simulink model "singledof_demo"  (Simulink 7.8)
settings: Solver=FixedStepDiscrete  StartTime=0.0  StopTime=inf  FixedStep=Ts  RelTol=1e-3
PreLoadFcn:
  | loadParametersSingleDof
InitFcn:
  | loadParametersSingleDof
values from neighbouring files (symbols this model uses):
  L_arm = 0.075    [freemot.mat]    (also in loadParametersSingleDof.m)
  lowOrder_tfd_foh = c2d(tf([1 2*pi*.64154],[1 0]),Ts,'foh')    [loadParametersSingleDof.m]
  maxTorque_allowed = 1.125    [freemot.mat]    (also in loadParametersSingleDof.m)
  torque_constant = 3.112    [freemot.mat]    (also in loadParametersSingleDof.m)
  Ts = 0.0005    [freemot.mat]
undefined symbols (not defined in the file or in its folder): DiscIntNeverNeededParam, shuntDynPredict_part1_tfd_foh, shuntDynPredict_part2_tfd_foh
libraries: simulink x32, simulink_extras x3
(part 2 of 2)

== system singledof_demo/AO DO/LED ==
  note: groen slave
      | rood slave
      |
      | groen master
      | rood master
  Logical Operator{6,8..10} (4 alike) : Logic  Operator=OR  AllPortsSameDT=off  OutDataTypeStr=boolean
  Logical Operator11 : Logic  AllPortsSameDT=off  OutDataTypeStr=boolean
  Logical Operator2 : Logic  AllPortsSameDT=off  OutDataTypeStr=boolean
  Logical Operator7 : Logic  Operator=NOT  AllPortsSameDT=off  OutDataTypeStr=boolean
  Mux1 : Mux
  LED : Outport
  wires:
  [tau_dm_saturated] -> Logical Operator11/2
  Logical Operator11/1 -> Logical Operator8/2
  Logical Operator2/1 -> Logical Operator6/2
  [tau_rm_saturated] -> Logical Operator10/2
  [tau_rs_saturated] -> Logical Operator9/2
  Logical Operator10/1 -> Mux1/4
  Logical Operator9/1 -> Mux1/2
  Logical Operator8/1 -> Mux1/3
  Logical Operator7/1 -> Logical Operator10/1, Logical Operator8/1, Logical Operator9/1, Logical Operator6/1
  [init_complete] -> Logical Operator7/1
  Logical Operator6/1 -> Mux1/1
  [tau_ds_saturated] -> Logical Operator2/2
  [Passivity_enable] -> Logical Operator11/1, Logical Operator2/1
  Mux1/1 -> LED/1

== system singledof_demo/AO DO/extraSafety ==
  V1 : Inport
  V2 : Inport  Port=2
  Abs : Abs
  Abs1 : Abs
  Compare To Constant : simulink/Logic and Bit Operations/Compare To Constant  relop=>  const=.5  OutDataTypeStr=uint8
  Compare To Constant1 : simulink/Logic and Bit Operations/Compare To Constant  relop=>  const=.5  OutDataTypeStr=uint8
  Logical Operator : Logic  Operator=OR  AllPortsSameDT=off  OutDataTypeStr=boolean
  Stop Simulation : Stop
  wires:
  Compare To Constant1/1 -> Logical Operator/2
  Compare To Constant/1 -> Logical Operator/1
  V2/1 -> Abs1/1
  V1/1 -> Abs/1
  Logical Operator/1 -> Stop Simulation/1
  Abs1/1 -> Compare To Constant1/1
  Abs/1 -> Compare To Constant/1

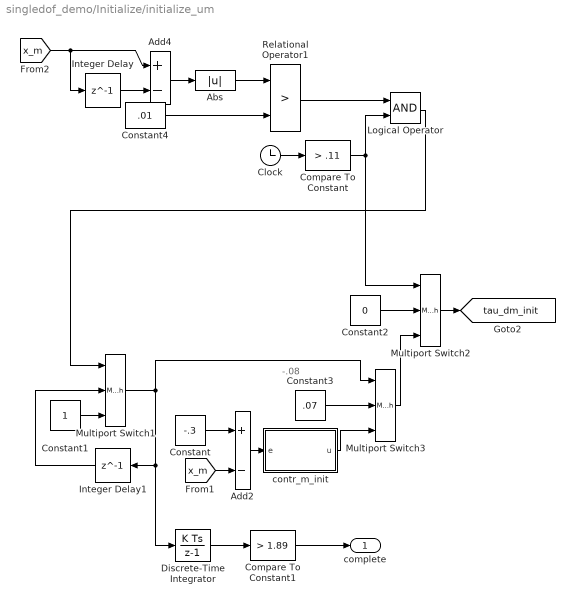
== system singledof_demo/Initialize/initialize_um ==
  note: -.08
  Abs : Abs
  Add2 : Sum  Inputs=+-
  Add4 : Sum  Inputs=+-
  Clock : Clock
  Compare To Constant : simulink/Logic and Bit Operations/Compare To Constant  relop=>  const=.11  OutDataTypeStr=uint8
  Compare To Constant1 : simulink/Logic and Bit Operations/Compare To Constant  relop=>  const=1.89  OutDataTypeStr=uint8
  Constant : Constant  Value=-.3
  Constant1 : Constant
  Constant2 : Constant  Value=0
  Constant3 : Constant  Value=.07
  Constant4 : Constant  Value=.01
  Discrete-Time Integrator : DiscreteIntegrator  SampleTime=Ts  ICPrevOutput=DiscIntNeverNeededParam  ICPrevScaledInput=DiscIntNeverNeededParam
  Integer Delay : Delay  DelayLength=1
  Integer Delay1 : Delay  DelayLength=1
  Logical Operator : Logic  AllPortsSameDT=off  OutDataTypeStr=boolean
  Multiport Switch1 : MultiPortSwitch  DataPortOrder=Zero-based contiguous  Inputs=2  zeroidx=on
  Multiport Switch2 : MultiPortSwitch  DataPortOrder=Zero-based contiguous  Inputs=2  zeroidx=on
  Multiport Switch3 : MultiPortSwitch  DataPortOrder=Zero-based contiguous  Inputs=2  zeroidx=on
  Relational Operator1 : RelationalOperator  Operator=>  OutDataTypeStr=boolean
  contr_m_init : Subsystem
      mask Display:
      | text(.1,.7,'Master')
      | text(.1,.3,'Controller')
  complete : Outport
  tag scope: tau_dm_init=global
  wires:
  Abs/1 -> Relational Operator1/1
  Constant2/1 -> Multiport Switch2/2
  Multiport Switch2/1 -> [tau_dm_init]
  Constant3/1 -> Multiport Switch3/2
  Multiport Switch3/1 -> Multiport Switch2/3
  contr_m_init/1(u) -> Multiport Switch3/3
  Compare To Constant1/1 -> complete/1
  Discrete-Time Integrator/1 -> Compare To Constant1/1
  Logical Operator/1 -> Multiport Switch1/1
  Compare To Constant/1 -> Multiport Switch2/1, Logical Operator/2
  Clock/1 -> Compare To Constant/1
  Relational Operator1/1 -> Logical Operator/1
  Add4/1 -> Abs/1
  [x_m] -> Integer Delay/1, Add4/1
  Constant4/1 -> Relational Operator1/2
  Integer Delay/1 -> Add4/2
  Constant/1 -> Add2/1
  Add2/1 -> contr_m_init/1(e)
  [x_m] -> Add2/2
  Constant1/1 -> Multiport Switch1/3
  Integer Delay1/1 -> Multiport Switch1/2
  Multiport Switch1/1 -> Multiport Switch3/1, Integer Delay1/1, Discrete-Time Integrator/1

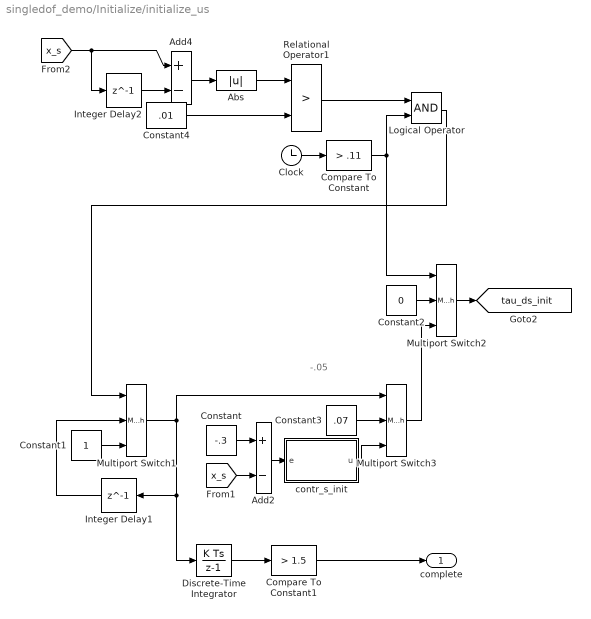
== system singledof_demo/Initialize/initialize_us ==
  note: -.05
  Abs : Abs
  Add2 : Sum  Inputs=+-
  Add4 : Sum  Inputs=+-
  Clock : Clock
  Compare To Constant : simulink/Logic and Bit Operations/Compare To Constant  relop=>  const=.11  OutDataTypeStr=uint8
  Compare To Constant1 : simulink/Logic and Bit Operations/Compare To Constant  relop=>  const=1.5  OutDataTypeStr=uint8
  Constant : Constant  Value=-.3
  Constant1 : Constant
  Constant2 : Constant  Value=0
  Constant3 : Constant  Value=.07
  Constant4 : Constant  Value=.01
  Discrete-Time Integrator : DiscreteIntegrator  SampleTime=Ts  ICPrevOutput=DiscIntNeverNeededParam  ICPrevScaledInput=DiscIntNeverNeededParam
  Integer Delay1 : Delay  DelayLength=1
  Integer Delay2 : Delay  DelayLength=1
  Logical Operator : Logic  AllPortsSameDT=off  OutDataTypeStr=boolean
  Multiport Switch1 : MultiPortSwitch  DataPortOrder=Zero-based contiguous  Inputs=2  zeroidx=on
  Multiport Switch2 : MultiPortSwitch  DataPortOrder=Zero-based contiguous  Inputs=2  zeroidx=on
  Multiport Switch3 : MultiPortSwitch  DataPortOrder=Zero-based contiguous  Inputs=2  zeroidx=on
  Relational Operator1 : RelationalOperator  Operator=>  OutDataTypeStr=boolean
  contr_s_init : Subsystem
      mask Display:
      | text(.1,.7,'Slave')
      | text(.1,.3,'Controller')
  complete : Outport
  tag scope: tau_ds_init=global
  wires:
  Abs/1 -> Relational Operator1/1
  Multiport Switch2/1 -> [tau_ds_init]
  Multiport Switch3/1 -> Multiport Switch2/3
  Constant2/1 -> Multiport Switch2/2
  contr_s_init/1(u) -> Multiport Switch3/3
  Constant3/1 -> Multiport Switch3/2
  Compare To Constant1/1 -> complete/1
  Discrete-Time Integrator/1 -> Compare To Constant1/1
  Multiport Switch1/1 -> Multiport Switch3/1, Integer Delay1/1, Discrete-Time Integrator/1
  Integer Delay1/1 -> Multiport Switch1/2
  Constant1/1 -> Multiport Switch1/3
  [x_s] -> Add2/2
  Add2/1 -> contr_s_init/1(e)
  Constant/1 -> Add2/1
  Integer Delay2/1 -> Add4/2
  Constant4/1 -> Relational Operator1/2
  [x_s] -> Integer Delay2/1, Add4/1
  Add4/1 -> Abs/1
  Relational Operator1/1 -> Logical Operator/1
  Clock/1 -> Compare To Constant/1
  Compare To Constant/1 -> Multiport Switch2/1, Logical Operator/2
  Logical Operator/1 -> Multiport Switch1/1

== system singledof_demo/Pos-force/contr_s ==
  e : Inport
  Add2 : Sum  Inputs=+++
  Discrete Derivative : simulink/Discrete/Discrete Derivative  gainval=1.0  ICPrevScaledInput=0.0  InputProcessing=Inherited  OutMin=[]  OutMax=[]  OutDataType=fixdt(1, 16)  OutScaling=2^-10  DoSatur=off
  Discrete-Time Integrator : DiscreteIntegrator  SampleTime=Ts  ICPrevOutput=DiscIntNeverNeededParam  ICPrevScaledInput=DiscIntNeverNeededParam
  Lowpass1 : Subsystem  mask{cf=100}
      mask prompts: cf "Cut off Frequency"
      mask help:
      | Discrete time first order lowpass filter, with cut-off frequency cf (Hz)
      | Kz / (z+K-1), with K=2*pi*cf*TS
      | For low frequencies this corresponds to the continous time lowpass filter
      | tf(1,[1/(2*pi*cf) 1])
      |
      | The maximum value for K=1, in this case output equals input
      | e.g. for 4000Hz sampling frequency the maximum value cf=4000/(2*pi)=637Hz.
      mask Display: text(.1,.5,['Lowpass @' num2str(cf) 'Hz'])
  P : Gain  Gain=Ps
  P1 : Gain  Gain=Is
  P2 : Gain  Gain=Ds
  anti windup : Subsystem
      mask Display: disp('anti-windup')
  u : Outport
  wires:
  Lowpass1/1(Out) -> P1/1, P2/1, P/1
  Add2/1 -> u/1, anti windup/2(contr output)
  P/1 -> Add2/1
  Discrete-Time Integrator/1 -> Add2/2
  P1/1 -> anti windup/1(In1)
  anti windup/1(Out1) -> Discrete-Time Integrator/1
  Discrete Derivative/1 -> Add2/3
  P2/1 -> Discrete Derivative/1
  e/1 -> Lowpass1/1(In)

== system singledof_demo/Pos-force/master to slave ==
  In1 : Inport
  Multiport Switch4 : MultiPortSwitch  DataPortOrder=Zero-based contiguous  Inputs=2  zeroidx=on
  TimeDelay1 : VariableTransportDelay  MaximumPoints=2000  FixedBuffer=on
  Unit Delay1 : UnitDelay  SampleTime=-1
  Out1 : Outport
  wires:
  Unit Delay1/1 -> Multiport Switch4/3
  TimeDelay1/1 -> Out1/1
  Multiport Switch4/1 -> Unit Delay1/1, TimeDelay1/1
  [comm_loss] -> Multiport Switch4/1
  [comm_delay] -> TimeDelay1/2
  In1/1 -> Multiport Switch4/2

== system singledof_demo/Pos-force/slave to master ==
  In1 : Inport
  Multiport Switch4 : MultiPortSwitch  DataPortOrder=Zero-based contiguous  Inputs=2  zeroidx=on
  TimeDelay1 : VariableTransportDelay  MaximumPoints=2000  FixedBuffer=on
  Unit Delay1 : UnitDelay  SampleTime=-1
  Out1 : Outport
  wires:
  Unit Delay1/1 -> Multiport Switch4/3
  TimeDelay1/1 -> Out1/1
  In1/1 -> Multiport Switch4/2
  [comm_delay] -> TimeDelay1/2
  [comm_loss] -> Multiport Switch4/1
  Multiport Switch4/1 -> Unit Delay1/1, TimeDelay1/1

== system singledof_demo/Pos-pos/contr_m ==
  e : Inport
  Add2 : Sum  Inputs=+++
  Discrete Derivative : simulink/Discrete/Discrete Derivative  gainval=1.0  ICPrevScaledInput=0.0  InputProcessing=Inherited  OutMin=[]  OutMax=[]  OutDataType=fixdt(1, 16)  OutScaling=2^-10  DoSatur=off
  Discrete-Time Integrator : DiscreteIntegrator  SampleTime=Ts  ICPrevOutput=DiscIntNeverNeededParam  ICPrevScaledInput=DiscIntNeverNeededParam
  Lowpass1 : Subsystem  mask{cf=100}
      mask prompts: cf "Cut off Frequency"
      mask help:
      | Discrete time first order lowpass filter, with cut-off frequency cf (Hz)
      | Kz / (z+K-1), with K=2*pi*cf*TS
      | For low frequencies this corresponds to the continous time lowpass filter
      | tf(1,[1/(2*pi*cf) 1])
      |
      | The maximum value for K=1, in this case output equals input
      | e.g. for 4000Hz sampling frequency the maximum value cf=4000/(2*pi)=637Hz.
      mask Display: text(.1,.5,['Lowpass @' num2str(cf) 'Hz'])
  P : Gain  Gain=Pm
  P1 : Gain  Gain=Im
  P2 : Gain  Gain=Dm
  anti windup : Subsystem
      mask Display: disp('anti-windup')
  u : Outport
  wires:
  Lowpass1/1(Out) -> P/1, P2/1, P1/1
  Add2/1 -> anti windup/2(contr output), u/1
  P/1 -> Add2/1
  Discrete-Time Integrator/1 -> Add2/2
  P1/1 -> anti windup/1(In1)
  anti windup/1(Out1) -> Discrete-Time Integrator/1
  Discrete Derivative/1 -> Add2/3
  P2/1 -> Discrete Derivative/1
  e/1 -> Lowpass1/1(In)

== system singledof_demo/Pos-pos/contr_s ==
  e : Inport
  Add2 : Sum  Inputs=+++
  Discrete Derivative : simulink/Discrete/Discrete Derivative  gainval=1.0  ICPrevScaledInput=0.0  InputProcessing=Inherited  OutMin=[]  OutMax=[]  OutDataType=fixdt(1, 16)  OutScaling=2^-10  DoSatur=off
  Discrete-Time Integrator : DiscreteIntegrator  SampleTime=Ts  ICPrevOutput=DiscIntNeverNeededParam  ICPrevScaledInput=DiscIntNeverNeededParam
  Lowpass1 : Subsystem  mask{cf=100}
      mask prompts: cf "Cut off Frequency"
      mask help:
      | Discrete time first order lowpass filter, with cut-off frequency cf (Hz)
      | Kz / (z+K-1), with K=2*pi*cf*TS
      | For low frequencies this corresponds to the continous time lowpass filter
      | tf(1,[1/(2*pi*cf) 1])
      |
      | The maximum value for K=1, in this case output equals input
      | e.g. for 4000Hz sampling frequency the maximum value cf=4000/(2*pi)=637Hz.
      mask Display: text(.1,.5,['Lowpass @' num2str(cf) 'Hz'])
  P : Gain  Gain=Ps
  P1 : Gain  Gain=Is
  P2 : Gain  Gain=Ds
  anti windup : Subsystem
      mask Display: disp('anti-windup')
  u : Outport
  wires:
  e/1 -> Lowpass1/1(In)
  P2/1 -> Discrete Derivative/1
  Discrete Derivative/1 -> Add2/3
  anti windup/1(Out1) -> Discrete-Time Integrator/1
  P1/1 -> anti windup/1(In1)
  Discrete-Time Integrator/1 -> Add2/2
  P/1 -> Add2/1
  Add2/1 -> anti windup/2(contr output), u/1
  Lowpass1/1(Out) -> P1/1, P2/1, P/1

== system singledof_demo/Pos-pos/master to slave ==
  In1 : Inport
  Multiport Switch4 : MultiPortSwitch  DataPortOrder=Zero-based contiguous  Inputs=2  zeroidx=on
  TimeDelay1 : VariableTransportDelay  MaximumPoints=2000  FixedBuffer=on
  Unit Delay1 : UnitDelay  SampleTime=-1
  Out1 : Outport
  wires:
  Unit Delay1/1 -> Multiport Switch4/3
  TimeDelay1/1 -> Out1/1
  Multiport Switch4/1 -> Unit Delay1/1, TimeDelay1/1
  [comm_loss] -> Multiport Switch4/1
  [comm_delay] -> TimeDelay1/2
  In1/1 -> Multiport Switch4/2

== system singledof_demo/Pos-pos/slave to master ==
  In1 : Inport
  Multiport Switch4 : MultiPortSwitch  DataPortOrder=Zero-based contiguous  Inputs=2  zeroidx=on
  TimeDelay1 : VariableTransportDelay  MaximumPoints=2000  FixedBuffer=on
  Unit Delay1 : UnitDelay  SampleTime=-1
  Out1 : Outport
  wires:
  Unit Delay1/1 -> Multiport Switch4/3
  TimeDelay1/1 -> Out1/1
  In1/1 -> Multiport Switch4/2
  [comm_delay] -> TimeDelay1/2
  [comm_loss] -> Multiport Switch4/1
  Multiport Switch4/1 -> Unit Delay1/1, TimeDelay1/1

== system singledof_demo/4channel (direct) OK/PD controller master/Lowpass1 ==
  In : Inport
  Constant1 : Constant
  Cut-off freq (Hz) : Constant  Value=cf
  Weighted Sample Time Math1 : SampleTimeMath  TsampMathOp=*
  lowpass : MATLAB Function  TreatAsAtomicUnit=on
  Out : Outport
  wires:
  Weighted Sample Time Math1/1 -> lowpass/3(Ts)
  Constant1/1 -> Weighted Sample Time Math1/1
  In/1 -> lowpass/1(in)
  lowpass/1(out) -> Out/1
  Cut-off freq (Hz)/1 -> lowpass/2(cf)

== system singledof_demo/4channel (direct) OK/PD controller slave/Lowpass1 ==
  In : Inport
  Constant1 : Constant
  Cut-off freq (Hz) : Constant  Value=cf
  Weighted Sample Time Math1 : SampleTimeMath  TsampMathOp=*
  lowpass : MATLAB Function  TreatAsAtomicUnit=on
  Out : Outport
  wires:
  Weighted Sample Time Math1/1 -> lowpass/3(Ts)
  Constant1/1 -> Weighted Sample Time Math1/1
  In/1 -> lowpass/1(in)
  lowpass/1(out) -> Out/1
  Cut-off freq (Hz)/1 -> lowpass/2(cf)

== system singledof_demo/AI DI/enc_master/EL5101 Encoder ==
  ec_EL5101_enc : S-Function  FunctionName=ec_EL5101_enc  Parameters=link_id  EnableBusSupport=off  mask{link_id=link_id}
      mask prompts: link_id "encoder in id (start from 1)"
  Out1 : Outport
  wires:
  ec_EL5101_enc/1 -> Out1/1

== system singledof_demo/AI DI/enc_master/EL5101 Latch ==
  ec_EL5101_enc : S-Function  FunctionName=ec_EL5101_latch  Parameters=link_id  EnableBusSupport=off  mask{link_id=link_id}
      mask prompts: link_id "encoder in id (start from 1)"
  Out1 : Outport
  wires:
  ec_EL5101_enc/1 -> Out1/1

== system singledof_demo/AI DI/enc_slave/EL5101 Encoder ==
  ec_EL5101_enc : S-Function  FunctionName=ec_EL5101_enc  Parameters=link_id  EnableBusSupport=off  mask{link_id=link_id}
      mask prompts: link_id "encoder in id (start from 1)"
  Out1 : Outport
  wires:
  ec_EL5101_enc/1 -> Out1/1

== system singledof_demo/AI DI/enc_slave/EL5101 Latch ==
  ec_EL5101_enc : S-Function  FunctionName=ec_EL5101_latch  Parameters=link_id  EnableBusSupport=off  mask{link_id=link_id}
      mask prompts: link_id "encoder in id (start from 1)"
  Out1 : Outport
  wires:
  ec_EL5101_enc/1 -> Out1/1

== system singledof_demo/AI DI/find_zero_during_init_m/moving avg ==
  force : Inport
  active : Inport  Port=2
  Add1 : Sum
  Add2 : Sum  Inputs=+-
  Add3 : Sum
  Integer Delay : Delay  DelayLength=1
  Integer Delay2 : Delay  DelayLength=1
  Multiport Switch2 : MultiPortSwitch  DataPortOrder=Zero-based contiguous  Inputs=2  zeroidx=on
  Product1 : Product  Inputs=*/  RndMeth=Zero
  Product2 : Product  Inputs=**  RndMeth=Zero
  constant : Constant  DisableCoverage=on
  constant1 : Constant  DisableCoverage=on
  constant2 : Constant  DisableCoverage=on
  avg : Outport
  wires:
  Product2/1 -> Add3/2
  Integer Delay2/1 -> Product2/1  "x(i-1)"
  Add2/1 -> Product2/2  "i-1"
  Product1/1 -> Integer Delay2/1, avg/1  "x(i)"
  Add3/1 -> Product1/1
  force/1 -> Add3/1  "a(i)"
  constant2/1 -> Add2/2
  Integer Delay/1 -> Add1/2
  constant1/1 -> Add1/1
  Multiport Switch2/1 -> Integer Delay/1, Product1/2, Add2/1  "i"
  Add1/1 -> Multiport Switch2/3
  constant/1 -> Multiport Switch2/2
  active/1 -> Multiport Switch2/1

== system singledof_demo/AI DI/find_zero_during_init_s/moving avg ==
  force : Inport
  active : Inport  Port=2
  Add1 : Sum
  Add2 : Sum  Inputs=+-
  Add3 : Sum
  Integer Delay : Delay  DelayLength=1
  Integer Delay1 : Delay  DelayLength=1
  Multiport Switch2 : MultiPortSwitch  DataPortOrder=Zero-based contiguous  Inputs=2  zeroidx=on
  Product1 : Product  Inputs=*/  RndMeth=Zero
  Product2 : Product  Inputs=**  RndMeth=Zero
  constant : Constant  DisableCoverage=on
  constant1 : Constant  DisableCoverage=on
  constant2 : Constant  DisableCoverage=on
  avg : Outport
  wires:
  active/1 -> Multiport Switch2/1
  constant/1 -> Multiport Switch2/2
  Add1/1 -> Multiport Switch2/3
  Multiport Switch2/1 -> Integer Delay/1, Add2/1, Product1/2  "i"
  constant1/1 -> Add1/1
  Integer Delay/1 -> Add1/2
  constant2/1 -> Add2/2
  force/1 -> Add3/1  "a(i)"
  Add3/1 -> Product1/1
  Product1/1 -> Integer Delay1/1, avg/1  "x(i)"
  Add2/1 -> Product2/2  "i-1"
  Integer Delay1/1 -> Product2/1  "x(i-1)"
  Product2/1 -> Add3/2

== system singledof_demo/Initialize/initialize_um/contr_m_init ==
  e : Inport
  Add2 : Sum  Inputs=+++
  D : simulink/Math Operations/Slider Gain  low=0  gain=0.05943  high=0.1
  Discrete Derivative : simulink/Discrete/Discrete Derivative  gainval=1.0  ICPrevScaledInput=0.0  InputProcessing=Inherited  OutMin=[]  OutMax=[]  OutDataType=fixdt(1, 16)  OutScaling=2^-10  DoSatur=off
  Discrete-Time Integrator : DiscreteIntegrator  SampleTime=Ts  ICPrevOutput=DiscIntNeverNeededParam  ICPrevScaledInput=DiscIntNeverNeededParam
  I : simulink/Math Operations/Slider Gain  low=0  gain=0.4692  high=1.637
  Lowpass3 : Subsystem  mask{cf=150}
      mask prompts: cf "Cut off Frequency"
      mask help:
      | Discrete time first order lowpass filter, with cut-off frequency cf (Hz)
      | Kz / (z+K-1), with K=2*pi*cf*TS
      | For low frequencies this corresponds to the continous time lowpass filter
      | tf(1,[1/(2*pi*cf) 1])
      |
      | The maximum value for K=1, in this case output equals input
      | e.g. for 4000Hz sampling frequency the maximum value cf=4000/(2*pi)=637Hz.
      mask Display: text(.1,.5,['Lowpass @' num2str(cf) 'Hz'])
  P : simulink/Math Operations/Slider Gain  low=0  gain=0.3734  high=0.6514
  anti windup : Subsystem
      mask Display: disp('anti-windup')
  u : Outport
  wires:
  e/1 -> P/1, I/1, D/1
  D/1 -> Lowpass3/1(In)
  Discrete Derivative/1 -> Add2/3
  anti windup/1(Out1) -> Discrete-Time Integrator/1
  I/1 -> anti windup/1(In1)
  Discrete-Time Integrator/1 -> Add2/2
  P/1 -> Add2/1
  Add2/1 -> anti windup/2(contr output), u/1
  Lowpass3/1(Out) -> Discrete Derivative/1

== system singledof_demo/Initialize/initialize_us/contr_s_init ==
  e : Inport
  Add2 : Sum  Inputs=+++
  D : simulink/Math Operations/Slider Gain  low=0  gain=0.05943  high=0.1
  Discrete Derivative : simulink/Discrete/Discrete Derivative  gainval=1.0  ICPrevScaledInput=0.0  InputProcessing=Inherited  OutMin=[]  OutMax=[]  OutDataType=fixdt(1, 16)  OutScaling=2^-10  DoSatur=off
  Discrete-Time Integrator : DiscreteIntegrator  SampleTime=Ts  ICPrevOutput=DiscIntNeverNeededParam  ICPrevScaledInput=DiscIntNeverNeededParam
  I : simulink/Math Operations/Slider Gain  low=0  gain=0.4692  high=1.637
  Lowpass3 : Subsystem  mask{cf=150}
      mask prompts: cf "Cut off Frequency"
      mask help:
      | Discrete time first order lowpass filter, with cut-off frequency cf (Hz)
      | Kz / (z+K-1), with K=2*pi*cf*TS
      | For low frequencies this corresponds to the continous time lowpass filter
      | tf(1,[1/(2*pi*cf) 1])
      |
      | The maximum value for K=1, in this case output equals input
      | e.g. for 4000Hz sampling frequency the maximum value cf=4000/(2*pi)=637Hz.
      mask Display: text(.1,.5,['Lowpass @' num2str(cf) 'Hz'])
  P : simulink/Math Operations/Slider Gain  low=0  gain=0.3734  high=0.6514
  anti windup : Subsystem
      mask Display: disp('anti-windup')
  u : Outport
  wires:
  Lowpass3/1(Out) -> Discrete Derivative/1
  Add2/1 -> u/1, anti windup/2(contr output)
  P/1 -> Add2/1
  Discrete-Time Integrator/1 -> Add2/2
  I/1 -> anti windup/1(In1)
  anti windup/1(Out1) -> Discrete-Time Integrator/1
  Discrete Derivative/1 -> Add2/3
  D/1 -> Lowpass3/1(In)
  e/1 -> D/1, I/1, P/1

== system singledof_demo/Pos-force/contr_s/Lowpass1 ==
  In : Inport
  Constant1 : Constant
  Cut-off freq (Hz) : Constant  Value=cf
  Weighted Sample Time Math1 : SampleTimeMath  TsampMathOp=*
  lowpass : MATLAB Function  TreatAsAtomicUnit=on
  Out : Outport
  wires:
  Weighted Sample Time Math1/1 -> lowpass/3(Ts)
  Constant1/1 -> Weighted Sample Time Math1/1
  In/1 -> lowpass/1(in)
  lowpass/1(out) -> Out/1
  Cut-off freq (Hz)/1 -> lowpass/2(cf)

== system singledof_demo/Pos-force/contr_s/anti windup ==
  In1 : Inport
  contr output : Inport  Port=2
  Ground : Ground
  Multiport Switch : MultiPortSwitch  DataPortOrder=Zero-based contiguous  Inputs=2  zeroidx=on
  Relational Operator : RelationalOperator  Operator===  OutDataTypeStr=boolean
  Out1 : Outport
  wires:
  Ground/1 -> Multiport Switch/2
  Relational Operator/1 -> Multiport Switch/1
  Multiport Switch/1 -> Out1/1
  In1/1 -> Multiport Switch/3
  contr output/1 -> Relational Operator/2
  [tau_rs] -> Relational Operator/1

== system singledof_demo/Pos-pos/contr_m/Lowpass1 ==
  In : Inport
  Constant1 : Constant
  Cut-off freq (Hz) : Constant  Value=cf
  Weighted Sample Time Math1 : SampleTimeMath  TsampMathOp=*
  lowpass : MATLAB Function  TreatAsAtomicUnit=on
  Out : Outport
  wires:
  Weighted Sample Time Math1/1 -> lowpass/3(Ts)
  Constant1/1 -> Weighted Sample Time Math1/1
  In/1 -> lowpass/1(in)
  lowpass/1(out) -> Out/1
  Cut-off freq (Hz)/1 -> lowpass/2(cf)

== system singledof_demo/Pos-pos/contr_m/anti windup ==
  In1 : Inport
  contr output : Inport  Port=2
  Ground : Ground
  Multiport Switch : MultiPortSwitch  DataPortOrder=Zero-based contiguous  Inputs=2  zeroidx=on
  Multiport Switch1 : MultiPortSwitch  DataPortOrder=Zero-based contiguous  Inputs=2  zeroidx=on
  Relational Operator : RelationalOperator  Operator===  OutDataTypeStr=boolean
  Sum1 : Sum  Inputs=+-
  Out1 : Outport
  wires:
  Relational Operator/1 -> Multiport Switch/1
  [F_TLC] -> Sum1/2
  Sum1/1 -> Multiport Switch1/3
  contr output/1 -> Sum1/1, Multiport Switch1/2
  [Passivity_enable] -> Multiport Switch1/1
  Multiport Switch1/1 -> Relational Operator/1
  [tau_rm] -> Relational Operator/2
  Ground/1 -> Multiport Switch/2
  Multiport Switch/1 -> Out1/1
  In1/1 -> Multiport Switch/3

== system singledof_demo/Pos-pos/contr_s/Lowpass1 ==
  In : Inport
  Constant1 : Constant
  Cut-off freq (Hz) : Constant  Value=cf
  Weighted Sample Time Math1 : SampleTimeMath  TsampMathOp=*
  lowpass : MATLAB Function  TreatAsAtomicUnit=on
  Out : Outport
  wires:
  Weighted Sample Time Math1/1 -> lowpass/3(Ts)
  Constant1/1 -> Weighted Sample Time Math1/1
  In/1 -> lowpass/1(in)
  lowpass/1(out) -> Out/1
  Cut-off freq (Hz)/1 -> lowpass/2(cf)

== system singledof_demo/Pos-pos/contr_s/anti windup ==
  In1 : Inport
  contr output : Inport  Port=2
  Ground : Ground
  Multiport Switch : MultiPortSwitch  DataPortOrder=Zero-based contiguous  Inputs=2  zeroidx=on
  Relational Operator : RelationalOperator  Operator===  OutDataTypeStr=boolean
  Out1 : Outport
  wires:
  Ground/1 -> Multiport Switch/2
  Relational Operator/1 -> Multiport Switch/1
  Multiport Switch/1 -> Out1/1
  In1/1 -> Multiport Switch/3
  contr output/1 -> Relational Operator/2
  [tau_rs] -> Relational Operator/1

== system singledof_demo/Initialize/initialize_um/contr_m_init/Lowpass3 ==
  In : Inport
  Constant1 : Constant
  Cut-off freq (Hz) : Constant  Value=cf
  Weighted Sample Time Math1 : SampleTimeMath  TsampMathOp=*
  lowpass : MATLAB Function  TreatAsAtomicUnit=on
  Out : Outport
  wires:
  Weighted Sample Time Math1/1 -> lowpass/3(Ts)
  Constant1/1 -> Weighted Sample Time Math1/1
  In/1 -> lowpass/1(in)
  lowpass/1(out) -> Out/1
  Cut-off freq (Hz)/1 -> lowpass/2(cf)

== system singledof_demo/Initialize/initialize_um/contr_m_init/anti windup ==
  In1 : Inport
  contr output : Inport  Port=2
  Ground : Ground
  Multiport Switch : MultiPortSwitch  DataPortOrder=Zero-based contiguous  Inputs=2  zeroidx=on
  Relational Operator : RelationalOperator  Operator===  OutDataTypeStr=boolean
  Out1 : Outport
  wires:
  [tau_rm] -> Relational Operator/1
  contr output/1 -> Relational Operator/2
  In1/1 -> Multiport Switch/3
  Multiport Switch/1 -> Out1/1
  Relational Operator/1 -> Multiport Switch/1
  Ground/1 -> Multiport Switch/2

== system singledof_demo/Initialize/initialize_us/contr_s_init/Lowpass3 ==
  In : Inport
  Constant1 : Constant
  Cut-off freq (Hz) : Constant  Value=cf
  Weighted Sample Time Math1 : SampleTimeMath  TsampMathOp=*
  lowpass : MATLAB Function  TreatAsAtomicUnit=on
  Out : Outport
  wires:
  Weighted Sample Time Math1/1 -> lowpass/3(Ts)
  Constant1/1 -> Weighted Sample Time Math1/1
  In/1 -> lowpass/1(in)
  lowpass/1(out) -> Out/1
  Cut-off freq (Hz)/1 -> lowpass/2(cf)

== system singledof_demo/Initialize/initialize_us/contr_s_init/anti windup ==
  In1 : Inport
  contr output : Inport  Port=2
  Ground : Ground
  Multiport Switch : MultiPortSwitch  DataPortOrder=Zero-based contiguous  Inputs=2  zeroidx=on
  Relational Operator : RelationalOperator  Operator===  OutDataTypeStr=boolean
  Out1 : Outport
  wires:
  Ground/1 -> Multiport Switch/2
  Relational Operator/1 -> Multiport Switch/1
  Multiport Switch/1 -> Out1/1
  In1/1 -> Multiport Switch/3
  contr output/1 -> Relational Operator/2
  [tau_rs] -> Relational Operator/1

== matlab function AI DI/Lowpass2/lowpass ==
  data: in input double; out output double; cf input double; Ts input double
function out  = fcn(in,cf,Ts)
% Discrete time first order lowpass filter, with cut-off frequency cf (Hz)
% Kz / (z+K-1), with K=2*pi*cf*TS
% For low frequencies this corresponds to the continous time lowpass filter
% tf(1,[1/(2*pi*cf) 1])
% 
% The maximum value for K=1, in this case output equals input
% e.g. for 4000Hz sampling frequency the maximum value cf=4000/(2*pi)=637Hz.
% 
% Beelen 2011

persistent out_prev
if isempty(out_prev)
    out_prev=zeros(size(in));
end

K=min(cf*2*pi*Ts,1); %Do not allow K to be bigger than 1...

out= out_prev + K* (in-out_prev);

out_prev=out;

== matlab function AI DI/Lowpass4/lowpass ==
  data: in input double; out output double; cf input double; Ts input double
function out  = fcn(in,cf,Ts)
% Discrete time first order lowpass filter, with cut-off frequency cf (Hz)
% Kz / (z+K-1), with K=2*pi*cf*TS
% For low frequencies this corresponds to the continous time lowpass filter
% tf(1,[1/(2*pi*cf) 1])
% 
% The maximum value for K=1, in this case output equals input
% e.g. for 4000Hz sampling frequency the maximum value cf=4000/(2*pi)=637Hz.
% 
% Beelen 2011

persistent out_prev
if isempty(out_prev)
    out_prev=zeros(size(in));
end

K=min(cf*2*pi*Ts,1); %Do not allow K to be bigger than 1...

out= out_prev + K* (in-out_prev);

out_prev=out;

== matlab function AI DI/Lowpass3/lowpass ==
  data: in input double; out output double; cf input double; Ts input double
function out  = fcn(in,cf,Ts)
% Discrete time first order lowpass filter, with cut-off frequency cf (Hz)
% Kz / (z+K-1), with K=2*pi*cf*TS
% For low frequencies this corresponds to the continous time lowpass filter
% tf(1,[1/(2*pi*cf) 1])
% 
% The maximum value for K=1, in this case output equals input
% e.g. for 4000Hz sampling frequency the maximum value cf=4000/(2*pi)=637Hz.
% 
% Beelen 2011

persistent out_prev
if isempty(out_prev)
    out_prev=zeros(size(in));
end

K=min(cf*2*pi*Ts,1); %Do not allow K to be bigger than 1...

out= out_prev + K* (in-out_prev);

out_prev=out;

== matlab function AI DI/Lowpass1/lowpass ==
  data: in input double; out output double; cf input double; Ts input double
function out  = fcn(in,cf,Ts)
% Discrete time first order lowpass filter, with cut-off frequency cf (Hz)
% Kz / (z+K-1), with K=2*pi*cf*TS
% For low frequencies this corresponds to the continous time lowpass filter
% tf(1,[1/(2*pi*cf) 1])
% 
% The maximum value for K=1, in this case output equals input
% e.g. for 4000Hz sampling frequency the maximum value cf=4000/(2*pi)=637Hz.
% 
% Beelen 2011

persistent out_prev
if isempty(out_prev)
    out_prev=zeros(size(in));
end

K=min(cf*2*pi*Ts,1); %Do not allow K to be bigger than 1...

out= out_prev + K* (in-out_prev);

out_prev=out;

== matlab function Initialize/initialize_um/contr_m_init/Lowpass3/lowpass ==
  data: in input double; out output double; cf input double; Ts input double
function out  = fcn(in,cf,Ts)
% Discrete time first order lowpass filter, with cut-off frequency cf (Hz)
% Kz / (z+K-1), with K=2*pi*cf*TS
% For low frequencies this corresponds to the continous time lowpass filter
% tf(1,[1/(2*pi*cf) 1])
% 
% The maximum value for K=1, in this case output equals input
% e.g. for 4000Hz sampling frequency the maximum value cf=4000/(2*pi)=637Hz.
% 
% Beelen 2011

persistent out_prev
if isempty(out_prev)
    out_prev=zeros(size(in));
end

K=min(cf*2*pi*Ts,1); %Do not allow K to be bigger than 1...

out= out_prev + K* (in-out_prev);

out_prev=out;

== matlab function Initialize/initialize_us/contr_s_init/Lowpass3/lowpass ==
  data: in input double; out output double; cf input double; Ts input double
function out  = fcn(in,cf,Ts)
% Discrete time first order lowpass filter, with cut-off frequency cf (Hz)
% Kz / (z+K-1), with K=2*pi*cf*TS
% For low frequencies this corresponds to the continous time lowpass filter
% tf(1,[1/(2*pi*cf) 1])
% 
% The maximum value for K=1, in this case output equals input
% e.g. for 4000Hz sampling frequency the maximum value cf=4000/(2*pi)=637Hz.
% 
% Beelen 2011

persistent out_prev
if isempty(out_prev)
    out_prev=zeros(size(in));
end

K=min(cf*2*pi*Ts,1); %Do not allow K to be bigger than 1...

out= out_prev + K* (in-out_prev);

out_prev=out;

== matlab function 4channel (direct) OK/PD controller slave/Lowpass1/lowpass ==
  data: in input double; out output double; cf input double; Ts input double
function out  = fcn(in,cf,Ts)
% Discrete time first order lowpass filter, with cut-off frequency cf (Hz)
% Kz / (z+K-1), with K=2*pi*cf*TS
% For low frequencies this corresponds to the continous time lowpass filter
% tf(1,[1/(2*pi*cf) 1])
% 
% The maximum value for K=1, in this case output equals input
% e.g. for 4000Hz sampling frequency the maximum value cf=4000/(2*pi)=637Hz.
% 
% Beelen 2011

persistent out_prev
if isempty(out_prev)
    out_prev=zeros(size(in));
end

K=min(cf*2*pi*Ts,1); %Do not allow K to be bigger than 1...

out= out_prev + K* (in-out_prev);

out_prev=out;

== matlab function 4channel (direct) OK/PD controller master/Lowpass1/lowpass ==
  data: in input double; out output double; cf input double; Ts input double
function out  = fcn(in,cf,Ts)
% Discrete time first order lowpass filter, with cut-off frequency cf (Hz)
% Kz / (z+K-1), with K=2*pi*cf*TS
% For low frequencies this corresponds to the continous time lowpass filter
% tf(1,[1/(2*pi*cf) 1])
% 
% The maximum value for K=1, in this case output equals input
% e.g. for 4000Hz sampling frequency the maximum value cf=4000/(2*pi)=637Hz.
% 
% Beelen 2011

persistent out_prev
if isempty(out_prev)
    out_prev=zeros(size(in));
end

K=min(cf*2*pi*Ts,1); %Do not allow K to be bigger than 1...

out= out_prev + K* (in-out_prev);

out_prev=out;

== matlab function Pos-pos/contr_m/Lowpass1/lowpass ==
  data: in input double; out output double; cf input double; Ts input double
function out  = fcn(in,cf,Ts)
% Discrete time first order lowpass filter, with cut-off frequency cf (Hz)
% Kz / (z+K-1), with K=2*pi*cf*TS
% For low frequencies this corresponds to the continous time lowpass filter
% tf(1,[1/(2*pi*cf) 1])
% 
% The maximum value for K=1, in this case output equals input
% e.g. for 4000Hz sampling frequency the maximum value cf=4000/(2*pi)=637Hz.
% 
% Beelen 2011

persistent out_prev
if isempty(out_prev)
    out_prev=zeros(size(in));
end

K=min(cf*2*pi*Ts,1); %Do not allow K to be bigger than 1...

out= out_prev + K* (in-out_prev);

out_prev=out;

== matlab function Pos-pos/contr_s/Lowpass1/lowpass ==
  data: in input double; out output double; cf input double; Ts input double
function out  = fcn(in,cf,Ts)
% Discrete time first order lowpass filter, with cut-off frequency cf (Hz)
% Kz / (z+K-1), with K=2*pi*cf*TS
% For low frequencies this corresponds to the continous time lowpass filter
% tf(1,[1/(2*pi*cf) 1])
% 
% The maximum value for K=1, in this case output equals input
% e.g. for 4000Hz sampling frequency the maximum value cf=4000/(2*pi)=637Hz.
% 
% Beelen 2011

persistent out_prev
if isempty(out_prev)
    out_prev=zeros(size(in));
end

K=min(cf*2*pi*Ts,1); %Do not allow K to be bigger than 1...

out= out_prev + K* (in-out_prev);

out_prev=out;

== matlab function Pos-force/contr_s/Lowpass1/lowpass ==
  data: in input double; out output double; cf input double; Ts input double
function out  = fcn(in,cf,Ts)
% Discrete time first order lowpass filter, with cut-off frequency cf (Hz)
% Kz / (z+K-1), with K=2*pi*cf*TS
% For low frequencies this corresponds to the continous time lowpass filter
% tf(1,[1/(2*pi*cf) 1])
% 
% The maximum value for K=1, in this case output equals input
% e.g. for 4000Hz sampling frequency the maximum value cf=4000/(2*pi)=637Hz.
% 
% Beelen 2011

persistent out_prev
if isempty(out_prev)
    out_prev=zeros(size(in));
end

K=min(cf*2*pi*Ts,1); %Do not allow K to be bigger than 1...

out= out_prev + K* (in-out_prev);

out_prev=out;
